simulink model "robArmDynamics"  (R2018b)
settings: Solver=VariableStepAuto  StartTime=0.0  StopTime=10.0  RelTol=1e-3
settings Model: Creator=Yahya  LastModifiedBy=Yahya

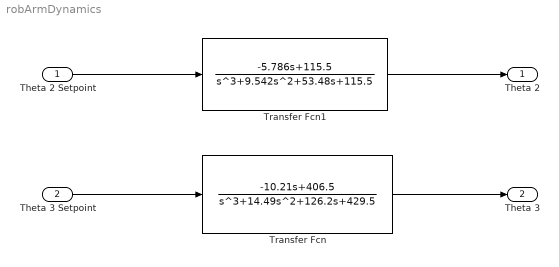
== system robArmDynamics ==
  Theta 2 Setpoint : Inport
  Theta 3 Setpoint : Inport  Port=2
  Transfer Fcn : TransferFcn  Numerator=[-10.21 406.5]  Denominator=[1 14.49 126.2 429.5]
  Transfer Fcn1 : TransferFcn  Numerator=[-5.786 115.5]  Denominator=[1 9.542 53.48 115.5]
  Theta 2 : Outport
  Theta 3 : Outport  Port=2
  wires:
  Theta 2 Setpoint/1 -> Transfer Fcn1/1
  Theta 3 Setpoint/1 -> Transfer Fcn/1
  Transfer Fcn1/1 -> Theta 2/1
  Transfer Fcn/1 -> Theta 3/1
